simulink model "LongitudinalVehicle"  (R2022b)
settings: Solver=VariableStepAuto  StartTime=0.0  StopTime=500  MaxStep=0.01  MinStep=1e-3  RelTol=1e-3
values from neighbouring files (symbols this model uses):
  contextModels =     [SimulinkContexts.mat]
libraries: HiL_Library x7
settings Model: DataDictionary=Library_Dictionary.sldd  Creator=niklas.baglikow  LastModifiedBy=niklas.baglikow

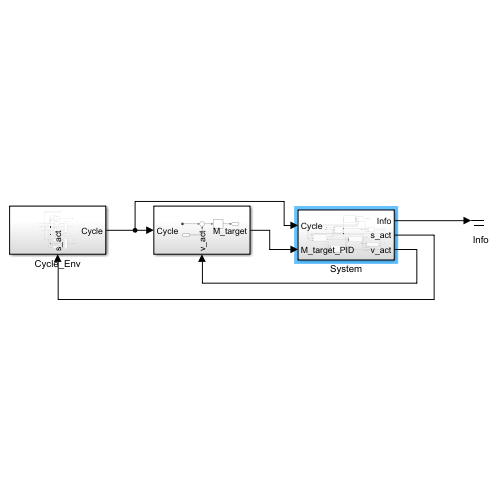
[thumbnail: Simulink's stored preview of the top-level diagram]
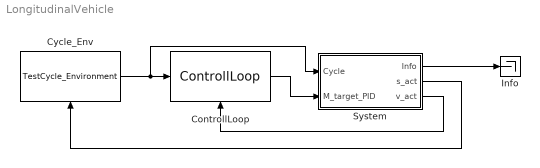
== system LongitudinalVehicle ==
  ControllLoop : HiL_Library/ControllLoop  SystemSampleTime=-1  VariantActivationTime=update diagram  Latency=0  AutoFrameSizeCalculation=off
      settings: SourceProductName=HiL Drivetrain Library  PortSchema="{\"entries\":[{\"content\":{\"sides\":[{\"content\":{\"connectorIds\":[\"In1\"]},\"type\":\"ConnectorPlacement.EquallySpacedRectSide\",\"uuid\":\"1335785d-f67d-41c9-8c38-7639e4454cfa\"},{\"content\":{\"connectorIds\":[\"Out1\"],\"side\":\"RIGHT\"},\"type\":\"ConnectorPlacement.EquallySpacedRectSide\",\"uuid\":\"0a417202-bd6c-4244-88bd-5f5b471a9f41\"},{\"content\":{\"side\":\"TOP\"},\"type\":\"ConnectorPlacement.EquallySpacedRectSide\",\"uuid\":\"7cab3c95-42cb-4345-89bc-9fe7f14c2d5b\"},{\"content\":{\"connectorIds\":[\"In2\"],\"side\":\"BOTTOM\"},\"type\":\"ConnectorPlacement.EquallySpacedRectSide\",\"uuid\":\"d4cd2bf5-131b-466c-8b33-e17efe7dc6cb\"}]},\"type\":\"ConnectorPlacement.EquallySpacedConnector\",\"uuid\":\"35880370-54ad-4605-8eb3-e99e84ebd17b\"}],\"packageUris\":[\"http://schema.mathworks.com/mf0/Connector/R2020b\"],\"version\":\"1.0\"}"
  Cycle_Env : HiL_Library/TestCycle_Environment  SystemSampleTime=-1  VariantActivationTime=update diagram  Latency=0  AutoFrameSizeCalculation=off
      settings: SourceProductName=HiL Drivetrain Library  PortSchema="{\"entries\":[{\"content\":{\"sides\":[{\"content\":{},\"type\":\"ConnectorPlacement.EquallySpacedRectSide\",\"uuid\":\"03033e87-b55c-4484-8c74-713d70ec0fa0\"},{\"content\":{\"connectorIds\":[\"Out1\"],\"side\":\"RIGHT\"},\"type\":\"ConnectorPlacement.EquallySpacedRectSide\",\"uuid\":\"8a89e092-682e-4192-8c28-bac37c8f3aca\"},{\"content\":{\"side\":\"TOP\"},\"type\":\"ConnectorPlacement.EquallySpacedRectSide\",\"uuid\":\"91e04554-c2cb-4814-b40c-a70d54db7d25\"},{\"content\":{\"connectorIds\":[\"In1\"],\"side\":\"BOTTOM\"},\"type\":\"ConnectorPlacement.EquallySpacedRectSide\",\"uuid\":\"04f7a2d7-0ce3-4cb0-a64f-2b57d8b48a0b\"}]},\"type\":\"ConnectorPlacement.EquallySpacedConnector\",\"uuid\":\"5260d7f7-6ac0-4054-8cf7-456fb5113596\"}],\"packageUris\":[\"http://schema.mathworks.com/mf0/Connector/R2020b\"],\"version\":\"1.0\"}"
  Info : Terminator
  System : Subsystem
  wires:
  Cycle_Env/1 -> ControllLoop/1, System/1(Cycle)
  ControllLoop/1 -> System/2(M_target_PID)
  System/1(Info) -> Info/1
  System/2(s_act) -> Cycle_Env/1
  System/3(v_act) -> ControllLoop/2

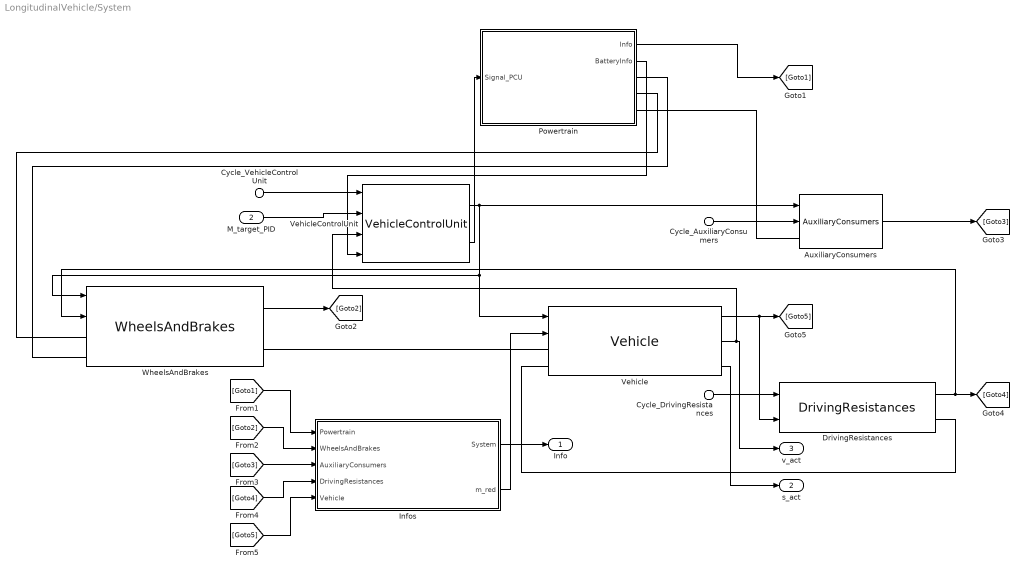
== system LongitudinalVehicle/System ==
  Cycle_AuxiliaryConsumers : Inport  PortName=Cycle
  Cycle_DrivingResistances : Inport  PortName=Cycle
  Cycle_VehicleControlUnit : Inport  PortName=Cycle
  M_target_PID : Inport  Port=2
  AuxiliaryConsumers : HiL_Library/AuxiliaryConsumers  P_Compressor=3200  P_Refrigerator=50  P_Radio=30  Day=0  P_Daytime_Running_Lights=14  P_Dipped_Beam=200  P_ElectricFan=400.83  P_ElectricCompressor=1704.6  TMS_conventionel=0  HV_Heating=HV_Heating  AirConditioning=AirConditioning
      settings: SourceProductName=HiL Drivetrain Library
  DrivingResistances : HiL_Library/DrivingResistances  g=9.81  f_r=0.007  c_w=0.53  A=10.2  rho_Air=1.204
      settings: SourceProductName=HiL Drivetrain Library
  Infos : Subsystem
  Powertrain : Subsystem  Variant=on
  Vehicle : HiL_Library/Vehicle  a_decel_limit=-5.51  m_tractor=11563  m_trailer=5875  m_max_total_allowed=contextModels(1).Parameters(7).Value  load_state=contextModels(1).Parameters(8).Value  mass_factor_gear1=3  mass_factor_gear2=1.2
      settings: SourceProductName=HiL Drivetrain Library
  VehicleControlUnit : HiL_Library/VehicleControlUnit  SystemSampleTime=-1  VariantActivationTime=update diagram  Latency=0  AutoFrameSizeCalculation=off
      settings: SourceProductName=HiL Drivetrain Library
  WheelsAndBrakes : HiL_Library/WheelsAndBrakes  d_w=1.0125  lambda=0.05  i_ges=-48.9886  J_red_Wheels=2.3322
      settings: SourceProductName=HiL Drivetrain Library
  Info : Outport
  s_act : Outport  Port=2
  v_act : Outport  Port=3
  wires:
  [Goto4] -> Infos/4(DrivingResistances)
  Cycle_VehicleControlUnit/1 -> VehicleControlUnit/1
  [Goto3] -> Infos/3(AuxiliaryConsumers)
  M_target_PID/1 -> VehicleControlUnit/2
  WheelsAndBrakes/1 -> [Goto2]
  [Goto1] -> Infos/1(Powertrain)
  Cycle_DrivingResistances/1 -> DrivingResistances/1
  [Goto2] -> Infos/2(WheelsAndBrakes)
  [Goto5] -> Infos/5(Vehicle)
  VehicleControlUnit/1 -> WheelsAndBrakes/1, Vehicle/1, AuxiliaryConsumers/1
  VehicleControlUnit/2 -> Powertrain/1(Signal_PCU)
  Infos/1(System) -> Info/1
  Infos/2(m_red) -> Vehicle/2
  Powertrain/1(Info) -> [Goto1]
  Vehicle/1 -> [Goto5], DrivingResistances/2
  Powertrain/2(BatteryInfo) -> VehicleControlUnit/4
  Vehicle/3 -> s_act/1
  Vehicle/2 -> VehicleControlUnit/3, v_act/1
  Cycle_AuxiliaryConsumers/1 -> AuxiliaryConsumers/2
  AuxiliaryConsumers/1 -> [Goto3]
  DrivingResistances/1 -> WheelsAndBrakes/2, [Goto4]
  connections:
  WheelsAndBrakes/RConn1 -- Vehicle/LConn1
  Powertrain/RConn2 -- WheelsAndBrakes/LConn1
  Powertrain/RConn3 -- AuxiliaryConsumers/LConn1
  Powertrain/RConn1 -- WheelsAndBrakes/LConn2
  DrivingResistances/RConn1 -- Vehicle/LConn2

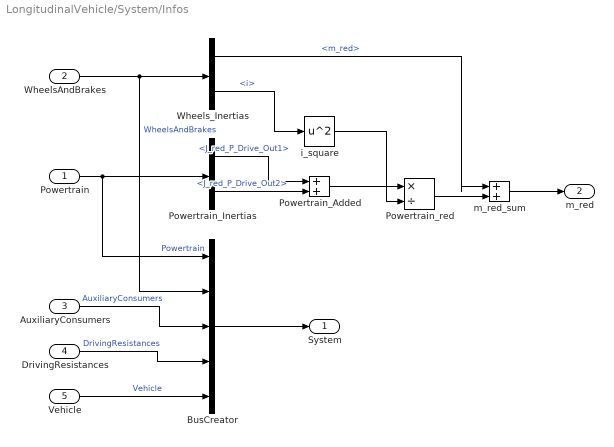
== system LongitudinalVehicle/System/Infos ==
  Powertrain : Inport
  WheelsAndBrakes : Inport  Port=2
  AuxiliaryConsumers : Inport  Port=3
  DrivingResistances : Inport  Port=4
  Vehicle : Inport  Port=5
  BusCreator : BusCreator  Inputs=5
  Powertrain_Added : Sum  Inputs=|++
  Powertrain_Inertias : BusSelector  OutputSignals=J_red_P_Drive_Out1,J_red_P_Drive_Out2
  Powertrain_red : Product  Inputs=*/
  Wheels_Inertias : BusSelector  OutputSignals=m_red,i
  i_square : Math  Operator=square
  m_red_sum : Sum  Inputs=|++
  System : Outport
  m_red : Outport  Port=2
  wires:
  WheelsAndBrakes/1 -> BusCreator/2, Wheels_Inertias/1  "WheelsAndBrakes"
  Powertrain_Inertias/1 -> Powertrain_Added/1  "<J_red_P_Drive_Out1>"
  Powertrain/1 -> BusCreator/1, Powertrain_Inertias/1  "Powertrain"
  Wheels_Inertias/1 -> m_red_sum/1  "<m_red>"
  AuxiliaryConsumers/1 -> BusCreator/3  "AuxiliaryConsumers"
  Wheels_Inertias/2 -> i_square/1  "<i>"
  DrivingResistances/1 -> BusCreator/4  "DrivingResistances"
  Vehicle/1 -> BusCreator/5  "Vehicle"
  Powertrain_Inertias/2 -> Powertrain_Added/2  "<J_red_P_Drive_Out2>"
  BusCreator/1 -> System/1
  i_square/1 -> Powertrain_red/2
  Powertrain_Added/1 -> Powertrain_red/1
  Powertrain_red/1 -> m_red_sum/2
  m_red_sum/1 -> m_red/1

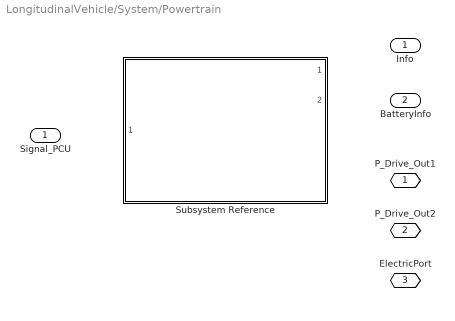
== system LongitudinalVehicle/System/Powertrain ==
  Signal_PCU : Inport  OutDataTypeStr=Bus: Signal_PCU
  Subsystem Reference : Subsystem  VariantControl=(default)  ReferencedSubsystem=PowertrainSubsystem
  P_Drive_Out1 : PMIOPort  Side=Right
  P_Drive_Out2 : PMIOPort  Port=2  Side=Right
  ElectricPort : PMIOPort  Port=3  Side=Right
  Info : Outport
  BatteryInfo : Outport  Port=2  OutDataTypeStr=Bus: Signal_Battery
